simulink model "PRBS_Signal_Generator"  (R2015a)
settings: Solver=ode45  StartTime=0.0  StopTime=10.0  RelTol=1e-3
libraries: simulink x1
settings Model: Creator=Yuri  LastModifiedBy=Yuri

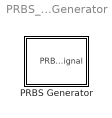
== system PRBS_Signal_Generator ==
  PRBS Generator : Subsystem

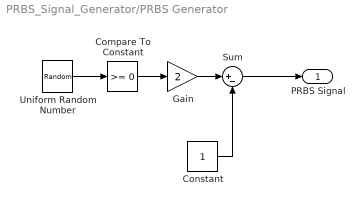
== system PRBS_Signal_Generator/PRBS Generator ==
  Compare To Constant : simulink/Logic and Bit Operations/Compare To Constant  relop=>=  const=0  OutDataTypeStr=boolean
  Constant : Constant
  Gain : Gain  Gain=2
  Sum : Sum  Inputs=|+-
  Uniform Random Number : UniformRandomNumber  SampleTime=0.1
  " PRBS Signal" : Outport
  wires:
  Uniform Random Number/1 -> Compare To Constant/1
  Compare To Constant/1 -> Gain/1
  Gain/1 -> Sum/1
  Sum/1 -> " PRBS Signal"/1
  Constant/1 -> Sum/2
